simulink model "Problem_2"  (R2020a)
settings: Solver=VariableStepAuto  StartTime=0.0  StopTime=inf  RelTol=1e-3
settings Model: Creator=Shubham Singh Rathor  LastModifiedBy=Shubham Singh Rathor

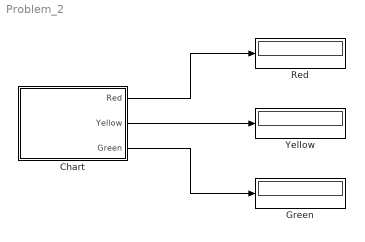
== system Problem_2 ==
  Chart : Stateflow chart  TreatAsAtomicUnit=on
  Green : Display
  Red : Display
  Yellow : Display
  wires:
  Chart/1(Red) -> Red/1
  Chart/2(Yellow) -> Yellow/1
  Chart/3(Green) -> Green/1

== stateflow chart Problem_2/Chart ==
  state Stop
    Red = 1;
    Yellow = 0;
    Green = 0;
  state Ready
    Red = 0;
    Yellow = 1;
    Green = 0;
  state Go
    Red = 0;
    Yellow = 0;
    Green = 1;
  state LaneChanging
    Red = 0;
    Yellow = 0;
    Green = 0;
  Stop -> Ready : after(20,sec)
  Ready -> Go : after(10,sec)
  LaneChanging -> Stop : after(20,sec)
  Go -> LaneChanging : after(10,sec)
  (default) -> LaneChanging
  data: Red output; Yellow output; Green output
